simulink model "EGRVlv_VDSens"  (R2016b)
settings: configuration reference "CodeGenConfigSet" (kept outside this file)
values from neighbouring files (symbols this model uses):
  EGRVlv_facAdapClsStrt_C = Calibration.Parameter    [init_EGRVlv_VDSens.m]
  EGRVlv_facAdapPosCls_C = Calibration.Parameter    [init_EGRVlv_VDSens.m]
  EGRVlv_facPT1_C = Calibration.Parameter    [init_EGRVlv_VDSens.m]
  EGRVlv_facPT1ModVal_C = Calibration.Parameter    [init_EGRVlv_VDSens.m]
  EGRVlv_IKiOfsLrnUp_C = Calibration.Parameter    [init_EGRVlv_VDSens.m]
  EGRVlv_numAdapClsMax_C = Calibration.Parameter    [init_EGRVlv_VDSens.m]
  EGRVlv_numEngTempOfsLrnRls1_C = Calibration.Parameter    [init_EGRVlv_VDSens.m]
  EGRVlv_numEngTempOfsLrnRls2_C = Calibration.Parameter    [init_EGRVlv_VDSens.m]
  EGRVlv_numTempSel_C = Calibration.Parameter    [init_EGRVlv_VDSens.m]
  EGRVlv_rActMax_C = Calibration.Parameter    [init_EGRVlv_VDSens.m]
  EGRVlv_rActMin_C = Calibration.Parameter    [init_EGRVlv_VDSens.m]
  EGRVlv_rActOfs_C = Calibration.Parameter    [init_EGRVlv_VDSens.m]
  EGRVlv_rAdapAgOpnMax_C = Calibration.Parameter    [init_EGRVlv_VDSens.m]
  EGRVlv_rAdapAgOpnMin_C = Calibration.Parameter    [init_EGRVlv_VDSens.m]
  EGRVlv_rAdapDiffPlaus_C = Calibration.Parameter    [init_EGRVlv_VDSens.m]
  EGRVlv_rAdapDiffPlausLgT_C = Calibration.Parameter    [init_EGRVlv_VDSens.m]
  EGRVlv_rAdapDiffPlausShT_C = Calibration.Parameter    [init_EGRVlv_VDSens.m]
  EGRVlv_rAdapIniOpn0_C = Calibration.Parameter    [init_EGRVlv_VDSens.m]
  EGRVlv_rAdapIniOpn_C = Calibration.Parameter    [init_EGRVlv_VDSens.m]
  EGRVlv_rAdapOpnBnd_C = Calibration.Parameter    [init_EGRVlv_VDSens.m]
  EGRVlv_rCmpNewCtlUn_C = Calibration.Parameter    [init_EGRVlv_VDSens.m]
  EGRVlv_RmpSlpNeg_C = Calibration.Parameter    [init_EGRVlv_VDSens.m]
  EGRVlv_RmpSlpPos_C = Calibration.Parameter    [init_EGRVlv_VDSens.m]
  EGRVlv_rOfsLrnDwn_C = Calibration.Parameter    [init_EGRVlv_VDSens.m]
  EGRVlv_rOfsLrnRmpDwnCls_C = Calibration.Parameter    [init_EGRVlv_VDSens.m]
  EGRVlv_rOfsLrnRmpUpFst_C = Calibration.Parameter    [init_EGRVlv_VDSens.m]
  EGRVlv_rOfsLrnVlvMax_C = Calibration.Parameter    [init_EGRVlv_VDSens.m]
  EGRVlv_rOfsLrnVlvMin_C = Calibration.Parameter    [init_EGRVlv_VDSens.m]
  EGRVlv_rOfsMax_C = Calibration.Parameter    [init_EGRVlv_VDSens.m]
  EGRVlv_rOfsMin_C = Calibration.Parameter    [init_EGRVlv_VDSens.m]
  EGRVlv_rPullDwnThres_C = Calibration.Parameter    [init_EGRVlv_VDSens.m]
  EGRVlv_rRmpDwnCls_C = Calibration.Parameter    [init_EGRVlv_VDSens.m]
  EGRVlv_rRmpUpFst_C = Calibration.Parameter    [init_EGRVlv_VDSens.m]
  EGRVlv_rSensVlvThres_C = Calibration.Parameter    [init_EGRVlv_VDSens.m]
  EGRVlv_rTmpOfsLrnMax_C = Calibration.Parameter    [init_EGRVlv_VDSens.m]
  EGRVlv_rTmpOfsLrnMin_C = Calibration.Parameter    [init_EGRVlv_VDSens.m]
  EGRVlv_rTransStgDfl_C = Calibration.Parameter    [init_EGRVlv_VDSens.m]
  EGRVlv_stNewVlvTrg_C = Calibration.Parameter    [init_EGRVlv_VDSens.m]
  EGRVlv_stOfsEngCond_C = Calibration.Parameter    [init_EGRVlv_VDSens.m]
  EGRVlv_stOfsLrnEnb_C = Calibration.Parameter    [init_EGRVlv_VDSens.m]
  EGRVlv_stOfsLrnTrg_C = Calibration.Parameter    [init_EGRVlv_VDSens.m]
  EGRVlv_swtActOfs_C = Calibration.Parameter    [init_EGRVlv_VDSens.m]
  EGRVlv_swtOfsLrnActv_C = Calibration.Parameter    [init_EGRVlv_VDSens.m]
  EGRVlv_swtSensPrs_C = Calibration.Parameter    [init_EGRVlv_VDSens.m]
  EGRVlv_tEngFldThresOfsLrnRls1_C = Calibration.Parameter    [init_EGRVlv_VDSens.m]
  EGRVlv_tEngFldThresOfsLrnRls2_C = Calibration.Parameter    [init_EGRVlv_VDSens.m]
  EGRVlv_tEngMax_C = Calibration.Parameter    [init_EGRVlv_VDSens.m]
  EGRVlv_tEngMin_C = Calibration.Parameter    [init_EGRVlv_VDSens.m]
  EGRVlv_tiAdapJamVlv_C = Calibration.Parameter    [init_EGRVlv_VDSens.m]
  EGRVlv_tiAdapWaitSensAcq_C = Calibration.Parameter    [init_EGRVlv_VDSens.m]
  EGRVlv_tiClsJamVlv_C = Calibration.Parameter    [init_EGRVlv_VDSens.m]
  EGRVlv_tiStable_C = Calibration.Parameter    [init_EGRVlv_VDSens.m]
  EGRVlv_uBattMax_C = Calibration.Parameter    [init_EGRVlv_VDSens.m]
  EGRVlv_uBattMin_C = Calibration.Parameter    [init_EGRVlv_VDSens.m]
  PRC_ZERO = fi(0,Prc_100_rate)    [init_EGRVlv_VDSens.m]
  SigTst_rEGRVlv_C = Calibration.Parameter    [init_EGRVlv_VDSens.m]
  SigTst_swtEGRVlv_C = Calibration.Parameter    [init_EGRVlv_VDSens.m]
undefined symbols (not defined in the file or in its folder): CEngDst_switch_conv, EGRVlv_VDSens_DT, EngState_conv, SubSysExeState_conv, Switch_conv
libraries: simulink x22, CXLib x18
(part 1 of 2)
settings Model: Creator=lvzhanghui  LastModifiedBy=zhulinfeng
settings ConfigSetRef: SourceLocation=Base Workspace

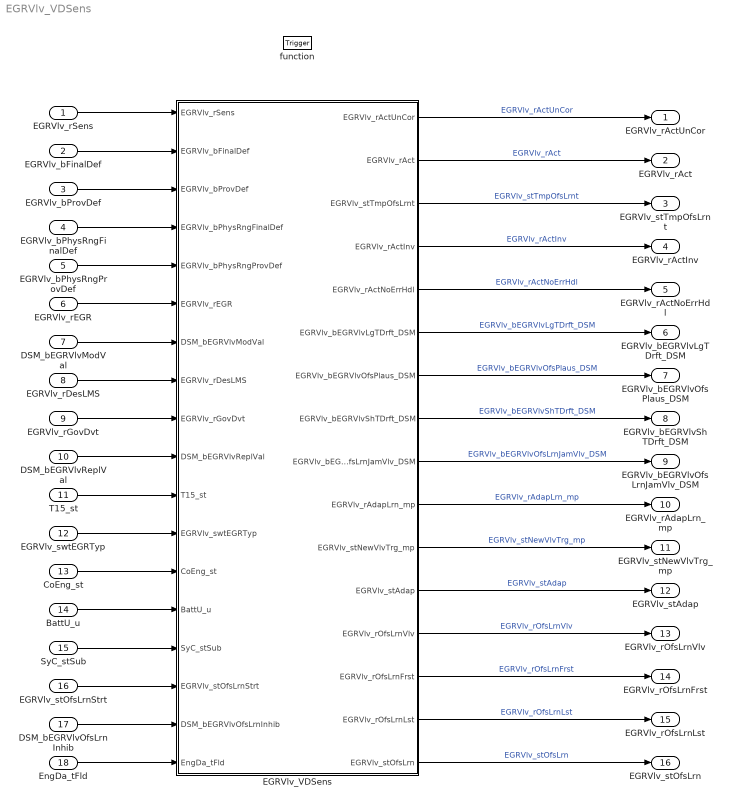
== system EGRVlv_VDSens ==
  EGRVlv_rSens : Inport  Tag=%  Description=Sensed value of actuator position without error handling  OutMin=-100  OutMax=100  OutDataTypeStr=Prc_100_rate
  EGRVlv_bFinalDef : Inport  Description=the final fault flag  Port=2  OutMin=0  OutMax=1  OutDataTypeStr=boolean
  EGRVlv_bProvDef : Inport  Description=the fault flag for the moment  Port=3  OutMin=0  OutMax=1  OutDataTypeStr=boolean
  EGRVlv_bPhysRngFinalDef : Inport  Description=Status Sensor of the EGR valve physical Signal range check finally defect  Port=4  OutMin=0  OutMax=1  OutDataTypeStr=boolean
  EGRVlv_bPhysRngProvDef : Inport  Description=Status Sensor of the EGR valve physical Signal range check temporary defect  Port=5  OutMin=0  OutMax=1  OutDataTypeStr=boolean
  EGRVlv_rEGR : Inport  Tag=%  Description=Control value for the EGR valve  Port=6  OutMin=-100  OutMax=100  OutDataTypeStr=Prc_100_rate
  DSM_bEGRVlvModVal : Inport  Description=Status of FId_EGRVlvModVal  Port=7  OutMin=0  OutMax=1  OutDataTypeStr=boolean
  EGRVlv_rDesLMS : Inport  Tag=%  Description=Desired value from LMS control  Port=8  OutMin=-100  OutMax=100  OutDataTypeStr=Prc_100_rate
  EGRVlv_rGovDvt : Inport  Tag=%  Description=Control deviation  Port=9  OutMin=-100  OutMax=100  OutDataTypeStr=Prc_100_rate
  DSM_bEGRVlvReplVal : Inport  Description=Status of FId_EGRVlvReplVal  Port=10  OutMin=0  OutMax=1  OutDataTypeStr=boolean
  T15_st : Inport  Description=Terminal 15 status after denouncing  Port=11  OutDataTypeStr=Enum: Switch_conv
  EGRVlv_swtEGRTyp : Inport  Description=Type of EGR actuator used  Port=12  OutMin=0  OutMax=255  OutDataTypeStr=State_uint8
  CoEng_st : Inport  Description=Engine coordinator state  Port=13  OutDataTypeStr=Enum: EngState_conv
  BattU_u : Inport  Tag=mv  Description=Battery voltage  Port=14  OutMin=0  OutMax=50000  OutDataTypeStr=Battery_mv
  SyC_stSub : Inport  Description=Current system/ECU sub-state  Port=15  OutDataTypeStr=Enum: SubSysExeState_conv
  EGRVlv_stOfsLrnStrt : Inport  Description=Diagnosis tester value to start offset learning  Port=16  OutMin=0  OutMax=1  OutDataTypeStr=boolean
  DSM_bEGRVlvOfsLrnInhib : Inport  Description=FId inhibited in case of system fault  Port=17  OutMin=0  OutMax=1  OutDataTypeStr=boolean
  EngDa_tFld : Inport  Tag=deg  Description=Engine temperature field  Port=18  OutMin=-3000  OutMax=3000  OutDataTypeStr=Temp_deg  PortDimensions=3
  function : TriggerPort  TriggerType=function-call  VariantControl=Variant
  EGRVlv_VDSens : Subsystem
  EGRVlv_rActUnCor : Outport  Tag=%  Description=Uncorrected position of the valve  OutMin=-100  OutMax=100  OutDataTypeStr=Prc_100_rate
  EGRVlv_rAct : Outport  Tag=%  Description=Actuatorposition  Port=2  OutMin=-100  OutMax=100  OutDataTypeStr=Prc_100_rate
  EGRVlv_stTmpOfsLrnt : Outport  Description=Temporary offset of the EGR valve is already learnt in the current driving cycle  Port=3  OutMin=0  OutMax=1  OutDataTypeStr=boolean
  EGRVlv_rActInv : Outport  Tag=%  Description=Actuatorposition (100% - rAct)  Port=4  OutMin=-100  OutMax=100  OutDataTypeStr=Prc_100_rate
  EGRVlv_rActNoErrHdl : Outport  Tag=%  Description=Valve position (offset corrected without error handling)  Port=5  OutMin=-100  OutMax=100  OutDataTypeStr=Prc_100_rate
  EGRVlv_bEGRVlvLgTDrft_DSM : Outport  Description=Fault path for long time valve drift  Port=6  OutMin=0  OutMax=1  OutDataTypeStr=boolean
  EGRVlv_bEGRVlvOfsPlaus_DSM : Outport  Description=Fault path for plausibility error  Port=7  OutMin=0  OutMax=1  OutDataTypeStr=boolean
  EGRVlv_bEGRVlvShTDrft_DSM : Outport  Description=Fault path for short time valve drift  Port=8  OutMin=0  OutMax=1  OutDataTypeStr=boolean
  EGRVlv_bEGRVlvOfsLrnJamVlv_DSM : Outport  Description=Fault path for jammed valve error during offset learning  Port=9  OutMin=0  OutMax=1  OutDataTypeStr=boolean
  EGRVlv_rAdapLrn_mp : Outport  Tag=%  Description=Offset learnt value in the present driving cycle  Port=10  OutMin=-100  OutMax=100  OutDataTypeStr=Prc_100_rate
  EGRVlv_stNewVlvTrg_mp : Outport  Description=New valve trigger status  Port=11  OutMin=0  OutMax=1  OutDataTypeStr=boolean
  EGRVlv_stAdap : Outport  Description=Status of offset learning  Port=12  OutMin=0  OutMax=65535  OutDataTypeStr=State_uint16
  EGRVlv_rOfsLrnVlv : Outport  Tag=%  Description=Control value for offset learning  Port=13  OutMin=-100  OutMax=100  OutDataTypeStr=Prc_100_rate
  EGRVlv_rOfsLrnFrst : Outport  Tag=%  Description=First learnt offset value stored in EEPROM  Port=14  OutMin=-100  OutMax=100  OutDataTypeStr=Prc_100_rate
  EGRVlv_rOfsLrnLst : Outport  Tag=%  Description=Last learnt offset value stored in EEPROM  Port=15  OutMin=-100  OutMax=100  OutDataTypeStr=Prc_100_rate
  EGRVlv_stOfsLrn : Outport  Description=Offset learning for Throttle valve complete  Port=16  OutMin=0  OutMax=255  OutDataTypeStr=State_uint8
  wires:
  EGRVlv_rSens/1 -> EGRVlv_VDSens/1(EGRVlv_rSens)
  EGRVlv_bFinalDef/1 -> EGRVlv_VDSens/2(EGRVlv_bFinalDef)
  EGRVlv_bProvDef/1 -> EGRVlv_VDSens/3(EGRVlv_bProvDef)
  EGRVlv_bPhysRngFinalDef/1 -> EGRVlv_VDSens/4(EGRVlv_bPhysRngFinalDef)
  EGRVlv_bPhysRngProvDef/1 -> EGRVlv_VDSens/5(EGRVlv_bPhysRngProvDef)
  EGRVlv_rEGR/1 -> EGRVlv_VDSens/6(EGRVlv_rEGR)
  DSM_bEGRVlvModVal/1 -> EGRVlv_VDSens/7(DSM_bEGRVlvModVal)
  EGRVlv_rDesLMS/1 -> EGRVlv_VDSens/8(EGRVlv_rDesLMS)
  EGRVlv_rGovDvt/1 -> EGRVlv_VDSens/9(EGRVlv_rGovDvt)
  DSM_bEGRVlvReplVal/1 -> EGRVlv_VDSens/10(DSM_bEGRVlvReplVal)
  T15_st/1 -> EGRVlv_VDSens/11(T15_st)
  EGRVlv_swtEGRTyp/1 -> EGRVlv_VDSens/12(EGRVlv_swtEGRTyp)
  CoEng_st/1 -> EGRVlv_VDSens/13(CoEng_st)
  BattU_u/1 -> EGRVlv_VDSens/14(BattU_u)
  SyC_stSub/1 -> EGRVlv_VDSens/15(SyC_stSub)
  EGRVlv_stOfsLrnStrt/1 -> EGRVlv_VDSens/16(EGRVlv_stOfsLrnStrt)
  DSM_bEGRVlvOfsLrnInhib/1 -> EGRVlv_VDSens/17(DSM_bEGRVlvOfsLrnInhib)
  EngDa_tFld/1 -> EGRVlv_VDSens/18(EngDa_tFld)
  EGRVlv_VDSens/1(EGRVlv_rActUnCor) -> EGRVlv_rActUnCor/1  "EGRVlv_rActUnCor"
  EGRVlv_VDSens/2(EGRVlv_rAct) -> EGRVlv_rAct/1  "EGRVlv_rAct"
  EGRVlv_VDSens/3(EGRVlv_stTmpOfsLrnt) -> EGRVlv_stTmpOfsLrnt/1  "EGRVlv_stTmpOfsLrnt"
  EGRVlv_VDSens/4(EGRVlv_rActInv) -> EGRVlv_rActInv/1  "EGRVlv_rActInv"
  EGRVlv_VDSens/5(EGRVlv_rActNoErrHdl) -> EGRVlv_rActNoErrHdl/1  "EGRVlv_rActNoErrHdl"
  EGRVlv_VDSens/6(EGRVlv_bEGRVlvLgTDrft_DSM) -> EGRVlv_bEGRVlvLgTDrft_DSM/1  "EGRVlv_bEGRVlvLgTDrft_DSM"
  EGRVlv_VDSens/7(EGRVlv_bEGRVlvOfsPlaus_DSM) -> EGRVlv_bEGRVlvOfsPlaus_DSM/1  "EGRVlv_bEGRVlvOfsPlaus_DSM"
  EGRVlv_VDSens/8(EGRVlv_bEGRVlvShTDrft_DSM) -> EGRVlv_bEGRVlvShTDrft_DSM/1  "EGRVlv_bEGRVlvShTDrft_DSM"
  EGRVlv_VDSens/9(EGRVlv_bEGRVlvOfsLrnJamVlv_DSM) -> EGRVlv_bEGRVlvOfsLrnJamVlv_DSM/1  "EGRVlv_bEGRVlvOfsLrnJamVlv_DSM"
  EGRVlv_VDSens/10(EGRVlv_rAdapLrn_mp) -> EGRVlv_rAdapLrn_mp/1  "EGRVlv_rAdapLrn_mp"
  EGRVlv_VDSens/11(EGRVlv_stNewVlvTrg_mp) -> EGRVlv_stNewVlvTrg_mp/1  "EGRVlv_stNewVlvTrg_mp"
  EGRVlv_VDSens/12(EGRVlv_stAdap) -> EGRVlv_stAdap/1  "EGRVlv_stAdap"
  EGRVlv_VDSens/13(EGRVlv_rOfsLrnVlv) -> EGRVlv_rOfsLrnVlv/1  "EGRVlv_rOfsLrnVlv"
  EGRVlv_VDSens/16(EGRVlv_stOfsLrn) -> EGRVlv_stOfsLrn/1  "EGRVlv_stOfsLrn"
  EGRVlv_VDSens/14(EGRVlv_rOfsLrnFrst) -> EGRVlv_rOfsLrnFrst/1  "EGRVlv_rOfsLrnFrst"
  EGRVlv_VDSens/15(EGRVlv_rOfsLrnLst) -> EGRVlv_rOfsLrnLst/1  "EGRVlv_rOfsLrnLst"

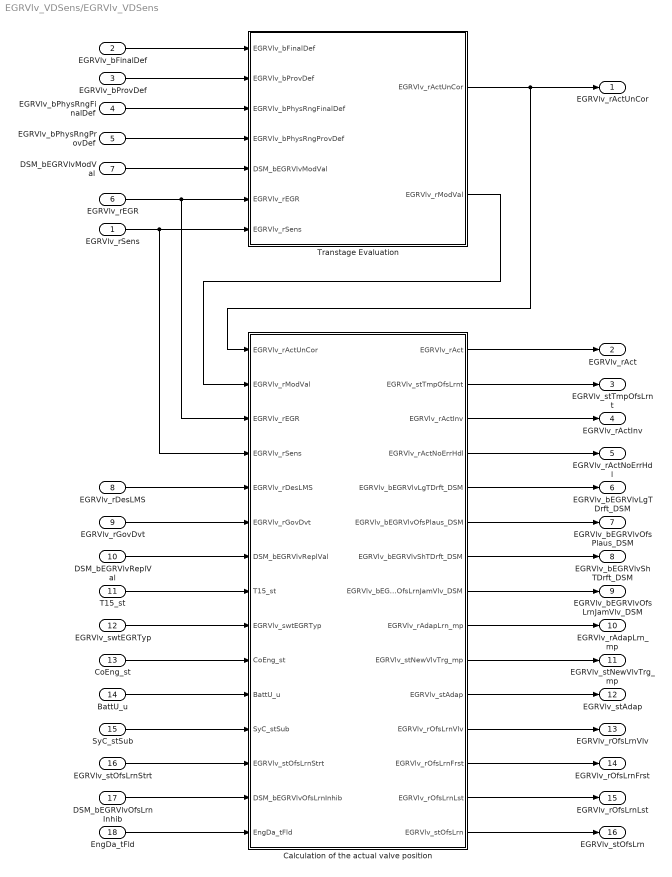
== system EGRVlv_VDSens/EGRVlv_VDSens ==
  EGRVlv_rSens : Inport  Tag=%
  EGRVlv_bFinalDef : Inport  Port=2
  EGRVlv_bProvDef : Inport  Port=3
  EGRVlv_bPhysRngFinalDef : Inport  Port=4
  EGRVlv_bPhysRngProvDef : Inport  Port=5
  EGRVlv_rEGR : Inport  Tag=%  Port=6
  DSM_bEGRVlvModVal : Inport  Tag=%  Port=7
  EGRVlv_rDesLMS : Inport  Port=8
  EGRVlv_rGovDvt : Inport  Port=9
  DSM_bEGRVlvReplVal : Inport  Tag=%  Port=10
  T15_st : Inport  Tag=%  Port=11
  EGRVlv_swtEGRTyp : Inport  Tag=%  Port=12
  CoEng_st : Inport  Port=13
  BattU_u : Inport  Tag=%  Port=14
  SyC_stSub : Inport  Tag=%  Port=15
  EGRVlv_stOfsLrnStrt : Inport  Tag=%  Port=16
  DSM_bEGRVlvOfsLrnInhib : Inport  Port=17
  EngDa_tFld : Inport  Tag=%  Port=18
  Calculation of the actual valve position : Subsystem
  Transtage Evaluation : Subsystem
  EGRVlv_rActUnCor : Outport  Tag=%
  EGRVlv_rAct : Outport  Tag=%  Port=2
  EGRVlv_stTmpOfsLrnt : Outport  Port=3
  EGRVlv_rActInv : Outport  Tag=%  Port=4
  EGRVlv_rActNoErrHdl : Outport  Port=5
  EGRVlv_bEGRVlvLgTDrft_DSM : Outport  Port=6
  EGRVlv_bEGRVlvOfsPlaus_DSM : Outport  Port=7
  EGRVlv_bEGRVlvShTDrft_DSM : Outport  Port=8
  EGRVlv_bEGRVlvOfsLrnJamVlv_DSM : Outport  Tag=%  Port=9
  EGRVlv_rAdapLrn_mp : Outport  Tag=%  Port=10
  EGRVlv_stNewVlvTrg_mp : Outport  Port=11
  EGRVlv_stAdap : Outport  Port=12
  EGRVlv_rOfsLrnVlv : Outport  Port=13
  EGRVlv_rOfsLrnFrst : Outport  Port=14
  EGRVlv_rOfsLrnLst : Outport  Port=15
  EGRVlv_stOfsLrn : Outport  Tag=%  Port=16
  wires:
  Transtage Evaluation/1(EGRVlv_rActUnCor) -> EGRVlv_rActUnCor/1, Calculation of the actual valve position/1(EGRVlv_rActUnCor)
  EGRVlv_rSens/1 -> Calculation of the actual valve position/4(EGRVlv_rSens), Transtage Evaluation/7(EGRVlv_rSens)
  EGRVlv_rEGR/1 -> Calculation of the actual valve position/3(EGRVlv_rEGR), Transtage Evaluation/6(EGRVlv_rEGR)
  Transtage Evaluation/2(EGRVlv_rModVal) -> Calculation of the actual valve position/2(EGRVlv_rModVal)
  EGRVlv_rDesLMS/1 -> Calculation of the actual valve position/5(EGRVlv_rDesLMS)
  EGRVlv_rGovDvt/1 -> Calculation of the actual valve position/6(EGRVlv_rGovDvt)
  DSM_bEGRVlvReplVal/1 -> Calculation of the actual valve position/7(DSM_bEGRVlvReplVal)
  T15_st/1 -> Calculation of the actual valve position/8(T15_st)
  EGRVlv_swtEGRTyp/1 -> Calculation of the actual valve position/9(EGRVlv_swtEGRTyp)
  CoEng_st/1 -> Calculation of the actual valve position/10(CoEng_st)
  BattU_u/1 -> Calculation of the actual valve position/11(BattU_u)
  SyC_stSub/1 -> Calculation of the actual valve position/12(SyC_stSub)
  EGRVlv_stOfsLrnStrt/1 -> Calculation of the actual valve position/13(EGRVlv_stOfsLrnStrt)
  DSM_bEGRVlvOfsLrnInhib/1 -> Calculation of the actual valve position/14(DSM_bEGRVlvOfsLrnInhib)
  EngDa_tFld/1 -> Calculation of the actual valve position/15(EngDa_tFld)
  EGRVlv_bFinalDef/1 -> Transtage Evaluation/1(EGRVlv_bFinalDef)
  EGRVlv_bProvDef/1 -> Transtage Evaluation/2(EGRVlv_bProvDef)
  EGRVlv_bPhysRngFinalDef/1 -> Transtage Evaluation/3(EGRVlv_bPhysRngFinalDef)
  EGRVlv_bPhysRngProvDef/1 -> Transtage Evaluation/4(EGRVlv_bPhysRngProvDef)
  DSM_bEGRVlvModVal/1 -> Transtage Evaluation/5(DSM_bEGRVlvModVal)
  Calculation of the actual valve position/1(EGRVlv_rAct) -> EGRVlv_rAct/1
  Calculation of the actual valve position/2(EGRVlv_stTmpOfsLrnt) -> EGRVlv_stTmpOfsLrnt/1
  Calculation of the actual valve position/3(EGRVlv_rActInv) -> EGRVlv_rActInv/1
  Calculation of the actual valve position/4(EGRVlv_rActNoErrHdl) -> EGRVlv_rActNoErrHdl/1
  Calculation of the actual valve position/5(EGRVlv_bEGRVlvLgTDrft_DSM) -> EGRVlv_bEGRVlvLgTDrft_DSM/1
  Calculation of the actual valve position/6(EGRVlv_bEGRVlvOfsPlaus_DSM) -> EGRVlv_bEGRVlvOfsPlaus_DSM/1
  Calculation of the actual valve position/7(EGRVlv_bEGRVlvShTDrft_DSM) -> EGRVlv_bEGRVlvShTDrft_DSM/1
  Calculation of the actual valve position/8(EGRVlv_bEGRVlvOfsLrnJamVlv_DSM) -> EGRVlv_bEGRVlvOfsLrnJamVlv_DSM/1
  Calculation of the actual valve position/9(EGRVlv_rAdapLrn_mp) -> EGRVlv_rAdapLrn_mp/1
  Calculation of the actual valve position/10(EGRVlv_stNewVlvTrg_mp) -> EGRVlv_stNewVlvTrg_mp/1
  Calculation of the actual valve position/11(EGRVlv_stAdap) -> EGRVlv_stAdap/1
  Calculation of the actual valve position/12(EGRVlv_rOfsLrnVlv) -> EGRVlv_rOfsLrnVlv/1
  Calculation of the actual valve position/13(EGRVlv_rOfsLrnFrst) -> EGRVlv_rOfsLrnFrst/1
  Calculation of the actual valve position/14(EGRVlv_rOfsLrnLst) -> EGRVlv_rOfsLrnLst/1
  Calculation of the actual valve position/15(EGRVlv_stOfsLrn) -> EGRVlv_stOfsLrn/1

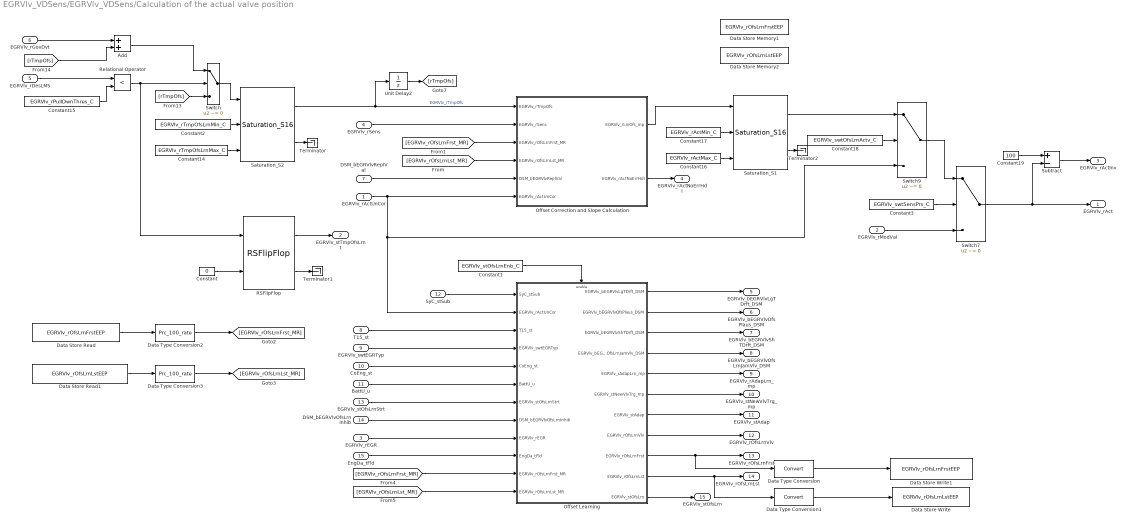
== system EGRVlv_VDSens/EGRVlv_VDSens/Calculation of the actual valve position ==
  EGRVlv_rActUnCor : Inport  Tag=%
  EGRVlv_rModVal : Inport  Tag=%  Port=2
  EGRVlv_rEGR : Inport  Tag=%  Port=3
  EGRVlv_rSens : Inport  Tag=%  Port=4
  EGRVlv_rDesLMS : Inport  Port=5
  EGRVlv_rGovDvt : Inport  Port=6
  DSM_bEGRVlvReplVal : Inport  Tag=%  Port=7
  T15_st : Inport  Tag=%  Port=8
  EGRVlv_swtEGRTyp : Inport  Tag=%  Port=9
  CoEng_st : Inport  Port=10
  BattU_u : Inport  Tag=%  Port=11
  SyC_stSub : Inport  Tag=%  Port=12
  EGRVlv_stOfsLrnStrt : Inport  Tag=%  Port=13
  DSM_bEGRVlvOfsLrnInhib : Inport  Port=14
  EngDa_tFld : Inport  Tag=%  Port=15
  Add : Sum  SaturateOnIntegerOverflow=on
  Constant : Constant  Value=0  OutDataTypeStr=boolean
  Constant1 : Constant  Value=EGRVlv_stOfsLrnEnb_C
  Constant14 : Constant  Value=EGRVlv_rTmpOfsLrnMax_C  SampleTime=-1
  Constant15 : Constant  Value=EGRVlv_rPullDwnThres_C  SampleTime=-1
  Constant16 : Constant  Value=EGRVlv_rActMax_C  SampleTime=-1
  Constant17 : Constant  Value=EGRVlv_rActMin_C  SampleTime=-1
  Constant18 : Constant  Value=EGRVlv_swtOfsLrnActv_C  SampleTime=-1
  Constant19 : Constant  Value=100  OutDataTypeStr=Prc_100_rate
  Constant2 : Constant  Value=EGRVlv_rTmpOfsLrnMin_C  SampleTime=-1
  Constant3 : Constant  Value=EGRVlv_swtSensPrs_C
  Data Store Memory1 : DataStoreMemory  DataStoreName=EGRVlv_rOfsLrnFrstEEP  ReadBeforeWriteMsg=warning  WriteAfterWriteMsg=warning  WriteAfterReadMsg=warning  ShowAdditionalParam=off  OutDataTypeStr=fixdt(1,16,100/8192,0)
  Data Store Memory2 : DataStoreMemory  DataStoreName=EGRVlv_rOfsLrnLstEEP  ReadBeforeWriteMsg=warning  WriteAfterWriteMsg=warning  WriteAfterReadMsg=warning  ShowAdditionalParam=off  OutDataTypeStr=fixdt(1,16,100/8192,0)
  Data Store Read : DataStoreRead  DataStoreName=EGRVlv_rOfsLrnFrstEEP
  Data Store Read1 : DataStoreRead  DataStoreName=EGRVlv_rOfsLrnLstEEP
  Data Store Write : DataStoreWrite  DataStoreName=EGRVlv_rOfsLrnLstEEP
  Data Store Write1 : DataStoreWrite  DataStoreName=EGRVlv_rOfsLrnFrstEEP
  Data Type Conversion : DataTypeConversion
  Data Type Conversion1 : DataTypeConversion
  Data Type Conversion2 : DataTypeConversion  OutDataTypeStr=Prc_100_rate
  Data Type Conversion3 : DataTypeConversion  OutDataTypeStr=Prc_100_rate
  Offset Correction and Slope Calculation : Subsystem
  Offset Learning : Subsystem
  RSFlipFlop : CXLib/RSFlipFlop
  Relational Operator : RelationalOperator  Operator=<  OutDataTypeStr=boolean  RndMeth=Simplest
  Saturation_S1 : CXLib/Saturation_S16
  Saturation_S2 : CXLib/Saturation_S16
  Subtract : Sum  Inputs=+-  SaturateOnIntegerOverflow=on
  Switch : Switch  Criteria=u2 ~= 0
  Switch7 : Switch  Criteria=u2 ~= 0  Threshold=CEngDst_switch_conv.OFF  InputSameDT=on
  Switch9 : Switch  Criteria=u2 ~= 0  Threshold=CEngDst_switch_conv.OFF  InputSameDT=on
  Terminator : Terminator
  Terminator1 : Terminator
  Terminator2 : Terminator
  Unit Delay2 : UnitDelay  SampleTime=-1
      settings: AttributesFormatString=InitialValue=%<InitialCondition>
  EGRVlv_rAct : Outport  Tag=%
  EGRVlv_stTmpOfsLrnt : Outport  Port=2
  EGRVlv_rActInv : Outport  Tag=%  Port=3
  EGRVlv_rActNoErrHdl : Outport  Port=4
  EGRVlv_bEGRVlvLgTDrft_DSM : Outport  Port=5
  EGRVlv_bEGRVlvOfsPlaus_DSM : Outport  Port=6
  EGRVlv_bEGRVlvShTDrft_DSM : Outport  Port=7
  EGRVlv_bEGRVlvOfsLrnJamVlv_DSM : Outport  Tag=%  Port=8
  EGRVlv_rAdapLrn_mp : Outport  Tag=%  Port=9
  EGRVlv_stNewVlvTrg_mp : Outport  Port=10
  EGRVlv_stAdap : Outport  Port=11
  EGRVlv_rOfsLrnVlv : Outport  Port=12
  EGRVlv_rOfsLrnFrst : Outport  Port=13
  EGRVlv_rOfsLrnLst : Outport  Port=14
  EGRVlv_stOfsLrn : Outport  Tag=%  Port=15
  wires:
  Constant3/1 -> Switch7/2
  Switch7/1 -> EGRVlv_rAct/1, Subtract/2
  Constant14/1 -> Saturation_S2/3
  Constant2/1 -> Saturation_S2/2
  Constant15/1 -> Relational Operator/2
  EGRVlv_rDesLMS/1 -> Relational Operator/1
  Relational Operator/1 -> RSFlipFlop/1, Switch/2
  EGRVlv_rGovDvt/1 -> Add/1
  Add/1 -> Switch/1
  [rTmpOfs] -> Switch/3
  Switch/1 -> Saturation_S2/1
  Saturation_S2/1 -> Offset Correction and Slope Calculation/1(EGRVlv_rTmpOfs), Unit Delay2/1  "EGRVlv_rTmpOfs"
  [rTmpOfs] -> Add/2
  Constant/1 -> RSFlipFlop/2
  Constant16/1 -> Saturation_S1/3
  Saturation_S1/1 -> Switch9/1
  Constant18/1 -> Switch9/2
  Constant17/1 -> Saturation_S1/2
  Switch9/1 -> Switch7/1
  Offset Correction and Slope Calculation/1(EGRVlv_rLinOfs_mp) -> Saturation_S1/1
  Constant19/1 -> Subtract/1
  Subtract/1 -> EGRVlv_rActInv/1
  Unit Delay2/1 -> [rTmpOfs]
  EGRVlv_rModVal/1 -> Switch7/3
  EGRVlv_rActUnCor/1 -> Offset Correction and Slope Calculation/6(EGRVlv_rActUnCor), Offset Learning/2(EGRVlv_rActUnCor), Switch9/3
  SyC_stSub/1 -> Offset Learning/1(SyC_stSub)
  EGRVlv_rSens/1 -> Offset Correction and Slope Calculation/2(EGRVlv_rSens)
  DSM_bEGRVlvReplVal/1 -> Offset Correction and Slope Calculation/5(DSM_bEGRVlvReplVal)
  T15_st/1 -> Offset Learning/3(T15_st)
  EGRVlv_swtEGRTyp/1 -> Offset Learning/4(EGRVlv_swtEGRTyp)
  CoEng_st/1 -> Offset Learning/5(CoEng_st)
  BattU_u/1 -> Offset Learning/6(BattU_u)
  EGRVlv_stOfsLrnStrt/1 -> Offset Learning/7(EGRVlv_stOfsLrnStrt)
  DSM_bEGRVlvOfsLrnInhib/1 -> Offset Learning/8(DSM_bEGRVlvOfsLrnInhib)
  EGRVlv_rEGR/1 -> Offset Learning/9(EGRVlv_rEGR)
  EngDa_tFld/1 -> Offset Learning/10(EngDa_tFld)
  [EGRVlv_rOfsLrnFrst_MR] -> Offset Learning/11(EGRVlv_rOfsLrnFrst_MR)
  [EGRVlv_rOfsLrnLst_MR] -> Offset Learning/12(EGRVlv_rOfsLrnLst_MR)
  Offset Correction and Slope Calculation/2(EGRVlv_rActNoErrHdl) -> EGRVlv_rActNoErrHdl/1
  Offset Learning/1(EGRVlv_bEGRVlvLgTDrft_DSM) -> EGRVlv_bEGRVlvLgTDrft_DSM/1
  Offset Learning/2(EGRVlv_bEGRVlvOfsPlaus_DSM) -> EGRVlv_bEGRVlvOfsPlaus_DSM/1
  Offset Learning/3(EGRVlv_bEGRVlvShTDrft_DSM) -> EGRVlv_bEGRVlvShTDrft_DSM/1
  Offset Learning/4(EGRVlv_bEGRVlvOfsLrnJamVlv_DSM) -> EGRVlv_bEGRVlvOfsLrnJamVlv_DSM/1
  Offset Learning/5(EGRVlv_rAdapLrn_mp) -> EGRVlv_rAdapLrn_mp/1
  Offset Learning/6(EGRVlv_stNewVlvTrg_mp) -> EGRVlv_stNewVlvTrg_mp/1
  Offset Learning/7(EGRVlv_stAdap) -> EGRVlv_stAdap/1
  Offset Learning/8(EGRVlv_rOfsLrnVlv) -> EGRVlv_rOfsLrnVlv/1
  RSFlipFlop/1 -> EGRVlv_stTmpOfsLrnt/1
  RSFlipFlop/2 -> Terminator1/1
  Saturation_S1/2 -> Terminator2/1
  Saturation_S2/2 -> Terminator/1
  Offset Learning/11(EGRVlv_stOfsLrn) -> EGRVlv_stOfsLrn/1
  Constant1/1 -> Offset Learning/Enable
  [EGRVlv_rOfsLrnLst_MR] -> Offset Correction and Slope Calculation/4(EGRVlv_rOfsLrnLst_MR)
  [EGRVlv_rOfsLrnFrst_MR] -> Offset Correction and Slope Calculation/3(EGRVlv_rOfsLrnFrst_MR)
  Data Store Read/1 -> Data Type Conversion2/1
  Data Store Read1/1 -> Data Type Conversion3/1
  Offset Learning/10(EGRVlv_rOfsLrnLst) -> Data Type Conversion1/1, EGRVlv_rOfsLrnLst/1
  Offset Learning/9(EGRVlv_rOfsLrnFrst) -> Data Type Conversion/1, EGRVlv_rOfsLrnFrst/1
  Data Type Conversion/1 -> Data Store Write1/1
  Data Type Conversion1/1 -> Data Store Write/1
  Data Type Conversion2/1 -> [EGRVlv_rOfsLrnFrst_MR]
  Data Type Conversion3/1 -> [EGRVlv_rOfsLrnLst_MR]

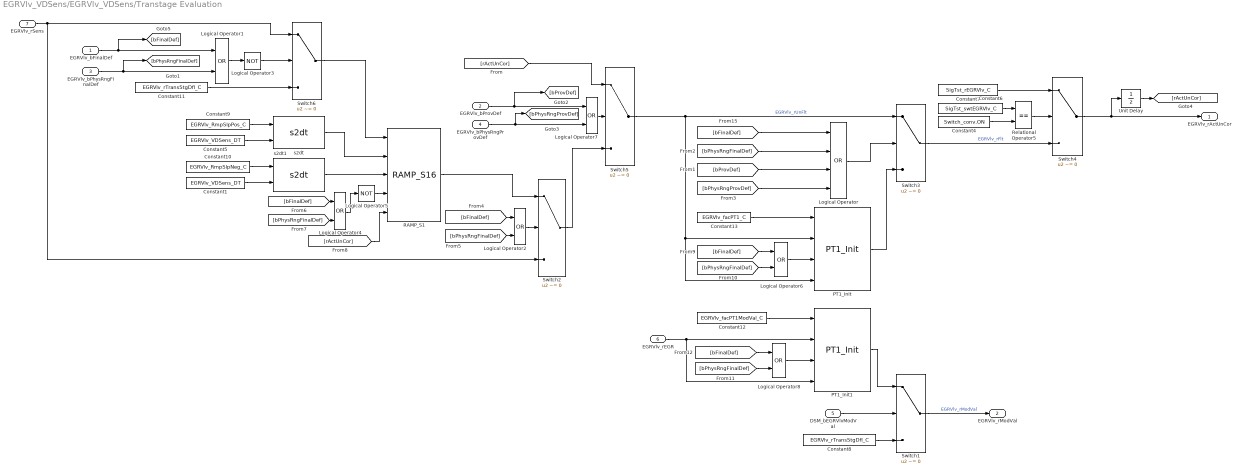
== system EGRVlv_VDSens/EGRVlv_VDSens/Transtage Evaluation ==
  EGRVlv_bFinalDef : Inport
  EGRVlv_bProvDef : Inport  Port=2
  EGRVlv_bPhysRngFinalDef : Inport  Port=3
  EGRVlv_bPhysRngProvDef : Inport  Port=4
  DSM_bEGRVlvModVal : Inport  Tag=%  Port=5
  EGRVlv_rEGR : Inport  Tag=%  Port=6
  EGRVlv_rSens : Inport  Tag=%  Port=7
  Constant1 : Constant  Value=EGRVlv_VDSens_DT
  Constant10 : Constant  Value=EGRVlv_RmpSlpNeg_C  SampleTime=-1
  Constant11 : Constant  Value=EGRVlv_rTransStgDfl_C  SampleTime=-1
  Constant12 : Constant  Value=EGRVlv_facPT1ModVal_C
  Constant13 : Constant  Value=EGRVlv_facPT1_C  SampleTime=-1
  Constant4 : Constant  Value=Switch_conv.ON
  Constant5 : Constant  Value=EGRVlv_VDSens_DT
  Constant6 : Constant  Value=SigTst_swtEGRVlv_C  SampleTime=-1
  Constant7 : Constant  Value=SigTst_rEGRVlv_C  SampleTime=-1
  Constant8 : Constant  Value=EGRVlv_rTransStgDfl_C
  Constant9 : Constant  Value=EGRVlv_RmpSlpPos_C  SampleTime=-1
  Logical Operator : Logic  Operator=OR  Inputs=4  OutDataTypeStr=boolean
  Logical Operator{1..2,4,6..8} (6 alike) : Logic  Operator=OR  OutDataTypeStr=boolean
  Logical Operator3 : Logic  Operator=NOT  AllPortsSameDT=off  OutDataTypeStr=boolean
  Logical Operator5 : Logic  Operator=NOT  AllPortsSameDT=off  OutDataTypeStr=boolean
  PT1_Init : CXLib/PT1_Init
  PT1_Init1 : CXLib/PT1_Init
  RAMP_S1 : CXLib/RAMP_S16
  Relational Operator5 : RelationalOperator  Operator===  OutDataTypeStr=boolean  RndMeth=Simplest  InputSameDT=on
  Switch1 : Switch  Criteria=u2 ~= 0  Threshold=CEngDst_switch_conv.OFF  InputSameDT=on
  Switch{2..3,5..6} (4 alike) : Switch  Criteria=u2 ~= 0  InputSameDT=on
  Switch4 : Switch  Criteria=u2 ~= 0  Threshold=CEngDst_switch_conv.OFF  InputSameDT=on
  Unit Delay : UnitDelay  SampleTime=-1
      settings: AttributesFormatString=InitialValue=%<InitialCondition>
  s2dt : CXLib/s2dt
  s2dt1 : CXLib/s2dt
  EGRVlv_rActUnCor : Outport  Tag=%
  EGRVlv_rModVal : Outport  Tag=%  Port=2
  wires:
  Constant6/1 -> Relational Operator5/1
  Logical Operator1/1 -> Logical Operator3/1
  Logical Operator3/1 -> Switch6/2
  Relational Operator5/1 -> Switch4/2
  [bPhysRngProvDef] -> Logical Operator/4
  [bPhysRngFinalDef] -> Logical Operator4/2
  Logical Operator5/1 -> RAMP_S1/4
  [rActUnCor] -> Switch5/1
  [bPhysRngFinalDef] -> Logical Operator6/2
  Constant5/1 -> s2dt/2
  [bFinalDef] -> Logical Operator2/1
  [bFinalDef] -> Logical Operator6/1
  Constant4/1 -> Relational Operator5/2
  s2dt1/1 -> RAMP_S1/3
  [bPhysRngFinalDef] -> Logical Operator2/2
  [bProvDef] -> Logical Operator/3
  s2dt/1 -> RAMP_S1/2
  [bPhysRngFinalDef] -> Logical Operator/2
  Logical Operator6/1 -> PT1_Init/3
  Constant1/1 -> s2dt1/2
  RAMP_S1/1 -> Switch2/1
  PT1_Init/1 -> Switch3/3
  Constant9/1 -> s2dt/1
  EGRVlv_bPhysRngProvDef/1 -> Logical Operator7/2, [bPhysRngProvDef]
  Logical Operator7/1 -> Switch5/2
  Logical Operator2/1 -> Switch2/2
  Logical Operator4/1 -> Logical Operator5/1
  Constant7/1 -> Switch4/1
  Switch6/1 -> RAMP_S1/1
  [bFinalDef] -> Logical Operator/1
  Unit Delay/1 -> [rActUnCor]
  EGRVlv_bFinalDef/1 -> Logical Operator1/1, [bFinalDef]
  Constant10/1 -> s2dt1/1
  EGRVlv_bPhysRngFinalDef/1 -> Logical Operator1/2, [bPhysRngFinalDef]
  Constant13/1 -> PT1_Init/1
  [bFinalDef] -> Logical Operator4/1
  EGRVlv_bProvDef/1 -> Logical Operator7/1, [bProvDef]
  Logical Operator/1 -> Switch3/2
  Constant11/1 -> Switch6/3
  EGRVlv_rSens/1 -> Switch6/1, Switch2/3
  Switch5/1 -> Switch3/1, PT1_Init/2, PT1_Init/4  "EGRVlv_rUnFlt"
  Switch3/1 -> Switch4/3  "EGRVlv_rFlt"
  Switch4/1 -> Unit Delay/1, EGRVlv_rActUnCor/1
  Switch2/1 -> Switch5/3
  DSM_bEGRVlvModVal/1 -> Switch1/2
  Switch1/1 -> EGRVlv_rModVal/1  "EGRVlv_rModVal"
  Constant8/1 -> Switch1/3
  PT1_Init1/1 -> Switch1/1
  EGRVlv_rEGR/1 -> PT1_Init1/2, PT1_Init1/4
  Constant12/1 -> PT1_Init1/1
  [bPhysRngFinalDef] -> Logical Operator8/2
  [bFinalDef] -> Logical Operator8/1
  Logical Operator8/1 -> PT1_Init1/3
  [rActUnCor] -> RAMP_S1/5

== system EGRVlv_VDSens/EGRVlv_VDSens/Calculation of the actual valve position/Offset Correction and Slope Calculation ==
  EGRVlv_rTmpOfs : Inport  Tag=%
  EGRVlv_rSens : Inport  Tag=%  Port=2
  EGRVlv_rOfsLrnFrst_MR : Inport  Tag=%  Port=3
  EGRVlv_rOfsLrnLst_MR : Inport  Tag=%  Port=4
  DSM_bEGRVlvReplVal : Inport  Tag=%  Port=5
  EGRVlv_rActUnCor : Inport  Tag=%  Port=6
  Add : Sum  SaturateOnIntegerOverflow=on
  Add1 : Sum  SaturateOnIntegerOverflow=on
  Add3 : Sum  SaturateOnIntegerOverflow=on
  Constant2 : Constant  Value=EGRVlv_rCmpNewCtlUn_C  SampleTime=-1
  Constant3 : Constant  Value=EGRVlv_swtActOfs_C  SampleTime=-1
  Constant4 : Constant  Value=EGRVlv_rActOfs_C  SampleTime=-1
  Logical Operator1 : Logic  Operator=OR  AllPortsSameDT=off  OutDataTypeStr=boolean
  Relational Operator1 : RelationalOperator  Operator===  OutDataTypeStr=boolean  RndMeth=Simplest
  Switch : Switch  Criteria=u2 ~= 0
  Switch1 : Switch  Criteria=u2 ~= 0
  EGRVlv_rLinOfs_mp : Outport
  EGRVlv_rActNoErrHdl : Outport  Port=2
  wires:
  EGRVlv_rSens/1 -> Add3/2
  EGRVlv_rTmpOfs/1 -> Add/2
  Switch/1 -> EGRVlv_rLinOfs_mp/1  "EGRVlv_rLinOfs_mp"
  Add3/1 -> EGRVlv_rActNoErrHdl/1
  DSM_bEGRVlvReplVal/1 -> Switch/2
  Constant2/1 -> Relational Operator1/2
  EGRVlv_rOfsLrnFrst_MR/1 -> Relational Operator1/1
  Relational Operator1/1 -> Logical Operator1/1
  Constant3/1 -> Logical Operator1/2
  Logical Operator1/1 -> Switch1/2
  EGRVlv_rOfsLrnLst_MR/1 -> Switch1/3
  Constant4/1 -> Switch1/1
  Add1/1 -> Add/1, Add3/1  "EGRVlv_rOfs_mp"
  Add/1 -> Switch/1
  Switch1/1 -> Add1/1
  EGRVlv_rActUnCor/1 -> Add1/2, Switch/3

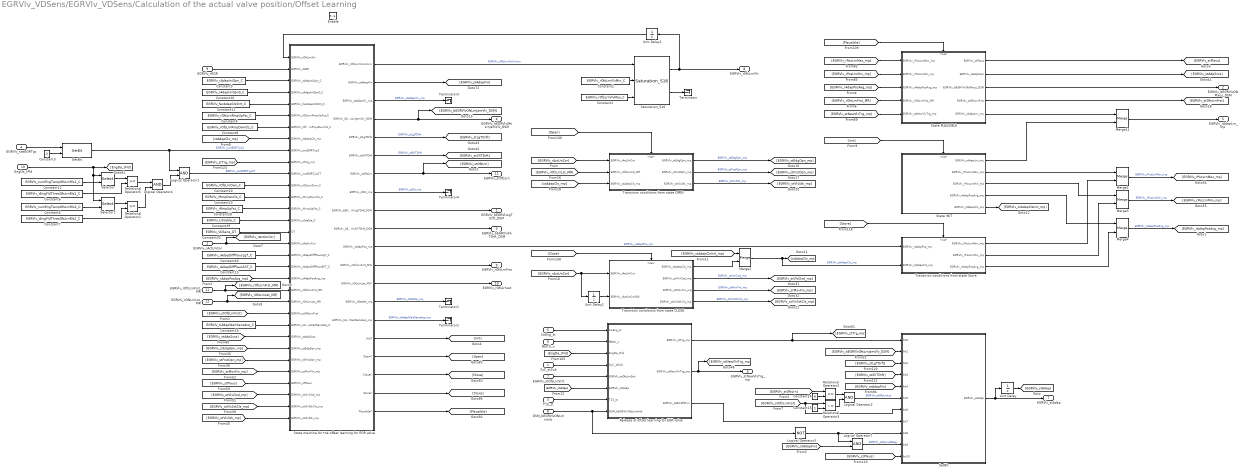
== system EGRVlv_VDSens/EGRVlv_VDSens/Calculation of the actual valve position/Offset Learning ==
  SyC_stSub : Inport  Tag=%
  EGRVlv_rActUnCor : Inport  Tag=%  Port=2
  T15_st : Inport  Tag=%  Port=3
  EGRVlv_swtEGRTyp : Inport  Tag=%  Port=4
  CoEng_st : Inport  Port=5
  BattU_u : Inport  Tag=%  Port=6
  EGRVlv_stOfsLrnStrt : Inport  Tag=%  Port=7
  DSM_bEGRVlvOfsLrnInhib : Inport  Port=8
  EGRVlv_rEGR : Inport  Tag=%  Port=9
  EngDa_tFld : Inport  Tag=%  Port=10
  EGRVlv_rOfsLrnFrst_MR : Inport  Tag=%  Port=11
  EGRVlv_rOfsLrnLst_MR : Inport  Tag=%  Port=12
  Enable : EnablePort
  Constant1 : Constant  Value=EGRVlv_rOfsLrnVlvMax_C
  Constant10 : Constant  Value=EGRVlv_rAdapIniOpn0_C
  Constant11 : Constant  Value=EGRVlv_facAdapClsStrt_C
  Constant12 : Constant  Value=EGRVlv_numEngTempOfsLrnRls1_C
  Constant13 : Constant  Value=EGRVlv_rAdapDiffPlausShT_C  SampleTime=-1
  Constant14 : Constant  Value=6  OutDataTypeStr=State_uint8
  Constant15 : Constant  OutDataTypeStr=State_uint8
  Constant16 : Constant  Value=EGRVlv_tiAdapWaitSensAcq_C  SampleTime=-1
  Constant2 : Constant  Value=EGRVlv_rOfsLrnVlvMin_C
  Constant20 : Constant  Value=EGRVlv_rOfsLrnDwn_C
  Constant23 : Constant  Value=EGRVlv_rRmpDwnCls_C
  Constant28 : Constant  Value=EGRVlv_rRmpUpFst_C
  Constant29 : Constant  Value=EGRVlv_tiStable_C
  Constant3 : Constant  Value=2  OutDataTypeStr=uint8
  Constant30 : Constant  Value=EGRVlv_VDSens_DT
  Constant4 : Constant  Value=EGRVlv_rOfsLrnRmpUpFst_C
  Constant40 : Constant  Value=EGRVlv_rAdapDiffPlausLgT_C  SampleTime=-1
  Constant5 : Constant  Value=EGRVlv_numEngTempOfsLrnRls2_C
  Constant6 : Constant  Value=EGRVlv_tEngFldThresOfsLrnRls1_C
  Constant7 : Constant  Value=EGRVlv_tEngFldThresOfsLrnRls2_C
  Constant8 : Constant  Value=EGRVlv_rOfsLrnRmpDwnCls_C
  Constant9 : Constant  Value=EGRVlv_rAdapIniOpn_C
  GetBit : CXLib/GetBit  dataTypeString=uint8  dataLength=0
      settings: AttributesFormatString=Get bit from %<dataTypeString>
  Logical Operator{1..2,4,7} (4 alike) : Logic  AllPortsSameDT=off  OutDataTypeStr=boolean
  Logical Operator3 : Logic  Operator=NOT  AllPortsSameDT=off  OutDataTypeStr=boolean
  Merge{1..4,11} (5 alike) : Merge
  Relational Operator1 : RelationalOperator  OutDataTypeStr=boolean  RndMeth=Simplest
  Relational Operator2 : RelationalOperator  Operator===  OutDataTypeStr=boolean  RndMeth=Simplest
  Relational Operator3 : RelationalOperator  Operator=~=  OutDataTypeStr=boolean  RndMeth=Simplest
  Relational Operator5 : RelationalOperator  OutDataTypeStr=boolean  RndMeth=Simplest
  Release of offset learning for EGR valve : Subsystem
  Saturation_S16 : CXLib/Saturation_S16
  Selector : Selector  IndexMode=Zero-based  InputPortWidth=3  IndexOptions=Index vector (port)  Indices=[1 3]  OutputSizes=1
  Selector1 : Selector  IndexMode=Zero-based  InputPortWidth=3  IndexOptions=Index vector (port)  Indices=[1 3]  OutputSizes=1
  SetBit : Subsystem
  State INIT : Subsystem  TreatAsAtomicUnit=on
  State PLAUSIBLE : Subsystem  TreatAsAtomicUnit=on
  State machine for the offset learning for EGR valve : Stateflow chart  TreatAsAtomicUnit=on
  Terminator{,1..4} (5 alike) : Terminator
  Transition conditions from state CLOSE : Subsystem  TreatAsAtomicUnit=on
  Transition conditions from state OPEN : Subsystem  TreatAsAtomicUnit=on
  Transition conditions from state Store : Subsystem
  Unit Delay : UnitDelay  SampleTime=-1
  Unit Delay1 : UnitDelay  SampleTime=-1
  Unit Delay2 : UnitDelay  SampleTime=-1
      settings: AttributesFormatString=InitialValue=%<InitialCondition>
  EGRVlv_bEGRVlvLgTDrft_DSM : Outport
  EGRVlv_bEGRVlvOfsPlaus_DSM : Outport  Port=2
  EGRVlv_bEGRVlvShTDrft_DSM : Outport  Port=3
  EGRVlv_bEGRVlvOfsLrnJamVlv_DSM : Outport  Tag=%  Port=4
  EGRVlv_rAdapLrn_mp : Outport  Tag=%  Port=5
  EGRVlv_stNewVlvTrg_mp : Outport  Port=6
  EGRVlv_stAdap : Outport  Port=7
  EGRVlv_rOfsLrnVlv : Outport  Port=8
  EGRVlv_rOfsLrnFrst : Outport  Port=9
  EGRVlv_rOfsLrnLst : Outport  Port=10
  EGRVlv_stOfsLrn : Outport  Tag=%  Port=11
  wires:
  Release of offset learning for EGR valve/1(EGRVlv_stTrg_mp) -> [EGRVlv_stTrg_mp], SetBit/1(bit0)
  Constant2/1 -> Saturation_S16/2
  Release of offset learning for EGR valve/3(EGRVlv_stBrkAftRun) -> SetBit/8(bit7)
  Merge11/1 -> EGRVlv_rAdapLrn_mp/1
  Release of offset learning for EGR valve/2(EGRVlv_stNewVlvTrg_mp) -> EGRVlv_stNewVlvTrg_mp/1, [EGRVlv_stNewVlvTrg_mp]
  Saturation_S16/1 -> EGRVlv_rOfsLrnVlv/1, Unit Delay1/1
  Constant1/1 -> Saturation_S16/3
  Constant5/1 -> Selector1/2
  Relational Operator5/1 -> Logical Operator4/1
  Logical Operator1/1 -> State machine for the offset learning for EGR valve/11(EGRVlv_swtEGRTyp2T)  "EGRVlv_swtEGRTyp2T"
  Logical Operator4/1 -> Logical Operator1/2
  Relational Operator1/1 -> Logical Operator4/2
  EGRVlv_rActUnCor/1 -> State machine for the offset learning for EGR valve/17(EGRVlv_rActUnCor), [EGRVlv_rActUnCor]
  Constant12/1 -> Selector/2
  EngDa_tFld/1 -> [EngDa_tFld], Selector/1, Selector1/1
  GetBit/1 -> State machine for the offset learning for EGR valve/9(EGRVlv_swtEGRTyp2), Logical Operator1/1  "EGRVlv_swtEGRTyp2"
  SetBit/1(EGRVlv_stAdap) -> EGRVlv_stAdap/1, Unit Delay/1
  Constant3/1 -> GetBit/2
  Selector/1 -> Relational Operator5/1
  State PLAUSIBLE/5(EGRVlv_rAdapLrn_mp) -> Merge11/1
  Constant7/1 -> Relational Operator1/2
  Constant6/1 -> Relational Operator5/2
  State INIT/1(EGRVlv_rAdapLrn_mp) -> Merge11/2
  Selector1/1 -> Relational Operator1/1
  [EGRVlv_stTrg_mp] -> State machine for the offset learning for EGR valve/10(EGRVlv_stTrg_mp)
  State machine for the offset learning for EGR valve/1(EGRVlv_rOfsLrnVlvUnLim) -> Saturation_S16/1  "EGRVlv_rOfsLrnVlvUnLim"
  Unit Delay/1 -> [EGRVlv_stAdap]
  [EGRVlv_stVlvStk_mp] -> State machine for the offset learning for EGR valve/32(EGRVlv_stVlvStk_mp)
  EGRVlv_swtEGRTyp/1 -> GetBit/1
  [EGRVlv_bEGRVlvOfsLrnJamVlv_DSM] -> SetBit/2(bit1)
  [EGRVlv_stLgTDrft] -> SetBit/3(bit2)
  [EGRVlv_stShTDrft] -> SetBit/4(bit3)
  [EGRVlv_stAdapFin] -> SetBit/5(bit4)
  Logical Operator2/1 -> SetBit/6(bit5)  "EGRVlv_stOfsLrnLst"
  Logical Operator7/1 -> SetBit/10(bit9)  "EGRVlv_stOpnLdDiag"
  [EGRVlv_stPlaus] -> SetBit/11(bit10)
  [EGRVlv_rPosLrnMax_mp] -> State PLAUSIBLE/1(EGRVlv_rPosLrnMax_mp)
  [EGRVlv_rPosLrnMin_mp] -> State PLAUSIBLE/2(EGRVlv_rPosLrnMin_mp)
  [EGRVlv_rAdapPosAvg_mp] -> State PLAUSIBLE/3(EGRVlv_rAdapPosAvg_mp)
  [EGRVlv_rOfsLrnFrst_MR] -> State PLAUSIBLE/4(EGRVlv_rOfsLrnFrst_MR)
  [EGRVlv_stNewVlvTrg_mp] -> State PLAUSIBLE/5(EGRVlv_stNewVlvTrg_mp)
  [Plausible] -> State PLAUSIBLE/Trigger
  [EGRVlv_rActUnCor] -> Unit Delay2/1, Transition conditions from state CLOSE/1(EGRVlv_rActUnCor)
  [Close] -> Transition conditions from state CLOSE/Trigger
  [EGRVlv_rOfsLrnLst_MR] -> Transition conditions from state OPEN/2(EGRVlv_rOfsLrnLst_MR)
  [ctAdapCls_mp] -> Transition conditions from state OPEN/3(EGRVlv_ctAdapCls_mp)
  [Open] -> Transition conditions from state OPEN/Trigger
  [Store] -> Transition conditions from state Store/Trigger
  Saturation_S16/2 -> Terminator/1
  State machine for the offset learning for EGR valve/9(EGRVlv_bEGRVlvLgTDrft_DSM) -> EGRVlv_bEGRVlvLgTDrft_DSM/1
  State PLAUSIBLE/3(EGRVlv_bEGRVlvOfsPlaus_DSM) -> EGRVlv_bEGRVlvOfsPlaus_DSM/1
  State machine for the offset learning for EGR valve/10(EGRVlv_bEGRVlvShTDrft_DSM) -> EGRVlv_bEGRVlvShTDrft_DSM/1
  State machine for the offset learning for EGR valve/3(EGRVlv_stAdapVlv_mp) -> Terminator3/1  "EGRVlv_stAdapVlv_mp"
  State machine for the offset learning for EGR valve/14(EGRVlv_tiStable_mp) -> Terminator1/1  "EGRVlv_tiStable_mp"
  State machine for the offset learning for EGR valve/11(EGRVlv_rAdapPos_mp) -> Transition conditions from state Store/1(EGRVlv_rAdapPos_mp)  "EGRVlv_rAdapPos_mp"
  State PLAUSIBLE/4(EGRVlv_stOfsLrnFrst) -> [EGRVlv_stOfsLrnFrst]
  Constant11/1 -> State machine for the offset learning for EGR valve/5(EGRVlv_facAdapClsStrt_C)
  Constant10/1 -> State machine for the offset learning for EGR valve/4(EGRVlv_rAdapIniOpn0_C)
  Constant9/1 -> State machine for the offset learning for EGR valve/3(EGRVlv_rAdapIniOpn_C)
  EGRVlv_rEGR/1 -> State machine for the offset learning for EGR valve/2(EGRVlv_rEGR)
  [EGRVlv_stVlvClsd_mp] -> State machine for the offset learning for EGR valve/30(EGRVlv_stVlvClsd_mp)
  [EGRVlv_stVlvStkCls_mp] -> State machine for the offset learning for EGR valve/31(EGRVlv_stVlvStkCls_mp)
  Constant8/1 -> State machine for the offset learning for EGR valve/7(EGRVlv_rOfsLrnRmpDwnCls_C)
  [EGRVlv_stMovFin_mp] -> State machine for the offset learning for EGR valve/28(EGRVlv_stMovFin_mp)
  Constant4/1 -> State machine for the offset learning for EGR valve/6(EGRVlv_rOfsLrnRmpUpFst_C)
  [EGRVlv_stFrstOpn_mp] -> State machine for the offset learning for EGR valve/27(EGRVlv_stFrstOpn_mp)
  [EGRVlv_stAdpSccs] -> State machine for the offset learning for EGR valve/25(EGRVlv_stAdpSccs)
  [EGRVlv_stEdgOpn_mp] -> State machine for the offset learning for EGR valve/26(EGRVlv_stEdgOpn_mp)
  [EGRVlv_stPlaus] -> State machine for the offset learning for EGR valve/29(EGRVlv_stPlaus)
  Constant20/1 -> State machine for the offset learning for EGR valve/12(EGRVlv_rOfsLrnDwn_C)
  Constant23/1 -> State machine for the offset learning for EGR valve/13(EGRVlv_rRmpDwnCls_C)
  Constant28/1 -> State machine for the offset learning for EGR valve/14(EGRVlv_rRmpUpFst_C)
  Constant29/1 -> State machine for the offset learning for EGR valve/15(EGRVlv_tiStable_C)
  Constant30/1 -> State machine for the offset learning for EGR valve/16(DT)
  [EGRVlv_stOfsLrnFrst] -> State machine for the offset learning for EGR valve/23(EGRVlv_stOfsLrnFrst)
  State machine for the offset learning for EGR valve/4(EGRVlv_bEGRVlvOfsLrnJamVlv_DSM) -> [EGRVlv_bEGRVlvOfsLrnJamVlv_DSM], EGRVlv_bEGRVlvOfsLrnJamVlv_DSM/1
  State machine for the offset learning for EGR valve/5(EGRVlv_stLgTDrft) -> [EGRVlv_stLgTDrft]  "EGRVlv_stLgTDrft"
  State machine for the offset learning for EGR valve/6(EGRVlv_stShTDrft) -> [EGRVlv_stShTDrft]  "EGRVlv_stShTDrft"
  State machine for the offset learning for EGR valve/7(EGRVlv_stOfsLrn) -> [EGRVlv_stOfsLrn], EGRVlv_stOfsLrn/1
  State machine for the offset learning for EGR valve/8(EGRVlv_stStr_mp) -> Terminator4/1  "EGRVlv_stStr_mp"
  State machine for the offset learning for EGR valve/2(EGRVlv_stAdapFin) -> [EGRVlv_stAdapFin]
  [EGRVlv_rActUnCor] -> Transition conditions from state OPEN/1(EGRVlv_rActUnCor)
  EGRVlv_rOfsLrnLst_MR/1 -> State machine for the offset learning for EGR valve/22(EGRVlv_rOfsLrnLst_MR), [EGRVlv_rOfsLrnLst_MR]
  EGRVlv_rOfsLrnFrst_MR/1 -> State machine for the offset learning for EGR valve/21(EGRVlv_rOfsLrnFrst_MR), [EGRVlv_rOfsLrnFrst_MR]
  [EGRVlv_rAdapPosAvg_mp] -> State machine for the offset learning for EGR valve/20(EGRVlv_rAdapPosAvg_mp)
  Constant13/1 -> State machine for the offset learning for EGR valve/19(EGRVlv_rAdapDiffPlausShT_C)
  Constant40/1 -> State machine for the offset learning for EGR valve/18(EGRVlv_rAdapDiffPlausLgT_C)
  State machine for the offset learning for EGR valve/13(EGRVlv_rOfsLrnLst_MW) -> EGRVlv_rOfsLrnLst/1
  State machine for the offset learning for EGR valve/15(EGRVlv_tiAdapWaitSensAcq_mp) -> Terminator2/1  "EGRVlv_tiAdapWaitSensAcq_mp"
  [EGRVlv_stAdapFin] -> Logical Operator7/2
  [EGRVlv_stOfsLrn] -> Relational Operator2/1
  Constant14/1 -> Relational Operator2/2
  [EGRVlv_stOfsLrnFrst] -> SetBit/7(bit6), Relational Operator3/1
  Constant15/1 -> Relational Operator3/2
  Relational Operator2/1 -> Logical Operator2/1
  Relational Operator3/1 -> Logical Operator2/2
  Constant16/1 -> State machine for the offset learning for EGR valve/24(EGRVlv_tiAdapWaitSensAcq_C)
  Logical Operator3/1 -> Logical Operator7/1, SetBit/9(bit8)
  Unit Delay1/1 -> State machine for the offset learning for EGR valve/1(EGRVlv_rOfsLrnVlv)
  [ctAdapCls_mp] -> State machine for the offset learning for EGR valve/8(EGRVlv_ctAdapCls_mp)
  Merge2/1 -> [EGRVlv_rPosLrnMax_mp]  "EGRVlv_rPosLrnMax_mp"
  Merge3/1 -> [EGRVlv_rPosLrnMin_mp]  "EGRVlv_rPosLrnMin_mp"
  Merge4/1 -> [EGRVlv_rAdapPosAvg_mp]  "EGRVlv_rAdapPosAvg_mp"
  State machine for the offset learning for EGR valve/17(Open()) -> [Open]
  State machine for the offset learning for EGR valve/18(Close()) -> [Close]
  State machine for the offset learning for EGR valve/19(Store()) -> [Store]
  State machine for the offset learning for EGR valve/20(Plausible()) -> [Plausible]
  Transition conditions from state OPEN/2(EGRVlv_stFrstOpn_mp) -> [EGRVlv_stFrstOpn_mp]  "EGRVlv_stFrstOpn_mp"
  Transition conditions from state OPEN/1(EGRVlv_stEdgOpn_mp) -> [EGRVlv_stEdgOpn_mp]  "EGRVlv_stEdgOpn_mp"
  Transition conditions from state OPEN/3(EGRVlv_stVlvStk_mp) -> [EGRVlv_stVlvStk_mp]  "EGRVlv_stVlvStk_mp"
  Transition conditions from state CLOSE/2(EGRVlv_stVlvClsd_mp) -> [EGRVlv_stVlvClsd_mp]  "EGRVlv_stVlvClsd_mp"
  Transition conditions from state CLOSE/3(EGRVlv_stMovFin_mp) -> [EGRVlv_stMovFin_mp]  "EGRVlv_stMovFin_mp"
  Transition conditions from state CLOSE/4(EGRVlv_stVlvStkCls_mp) -> [EGRVlv_stVlvStkCls_mp]  "EGRVlv_stVlvStkCls_mp"
  State PLAUSIBLE/2(EGRVlv_stAdpSccs) -> [EGRVlv_stAdpSccs]
  State machine for the offset learning for EGR valve/16(Init()) -> [Init]
  [Init] -> State INIT/Trigger
  Merge1/1 -> Transition conditions from state Store/2(EGRVlv_ctAdapCls_mp), [ctAdapCls_mp]  "EGRVlv_ctAdapCls_mp"
  Transition conditions from state CLOSE/1(EGRVlv_ctAdapCls_mp) -> Merge1/2
  State INIT/2(EGRVlv_rPosLrnMax_mp) -> Merge2/1
  State INIT/3(EGRVlv_rPosLrnMin_mp) -> Merge3/1
  State INIT/4(EGRVlv_rAdapPosAvg_mp) -> Merge4/1
  State INIT/5(EGRVlv_ctAdapCls_mp) -> [EGRVlv_ctAdapClsInit_mp]
  [EGRVlv_ctAdapClsInit_mp] -> Merge1/1
  Transition conditions from state Store/1(EGRVlv_rPosLrnMax_mp) -> Merge2/2
  Transition conditions from state Store/2(EGRVlv_rPosLrnMin_mp) -> Merge3/2
  Transition conditions from state Store/3(EGRVlv_rAdapPosAvg_mp) -> Merge4/2
  Unit Delay2/1 -> Transition conditions from state CLOSE/2(EGRVlv_rActUnCorOld)
  State PLAUSIBLE/1(EGRVlv_stPlaus) -> [EGRVlv_stPlaus]
  DSM_bEGRVlvOfsLrnInhib/1 -> Logical Operator3/1, Release of offset learning for EGR valve/8(DSM_bEGRVlvOfsLrnInhib)
  CoEng_st/1 -> Release of offset learning for EGR valve/1(CoEng_st)
  BattU_u/1 -> Release of offset learning for EGR valve/2(BattU_u)
  [EngDa_tFld] -> Release of offset learning for EGR valve/3(EngDa_tFld)
  SyC_stSub/1 -> Release of offset learning for EGR valve/4(SyC_stSub)
  EGRVlv_stOfsLrnStrt/1 -> Release of offset learning for EGR valve/5(EGRVlv_stOfsLrnStrt)
  [EGRVlv_stAdap] -> Release of offset learning for EGR valve/6(EGRVlv_stAdap)
  T15_st/1 -> Release of offset learning for EGR valve/7(T15_st)
  State machine for the offset learning for EGR valve/12(EGRVlv_rOfsLrnFrst_MW) -> EGRVlv_rOfsLrnFrst/1

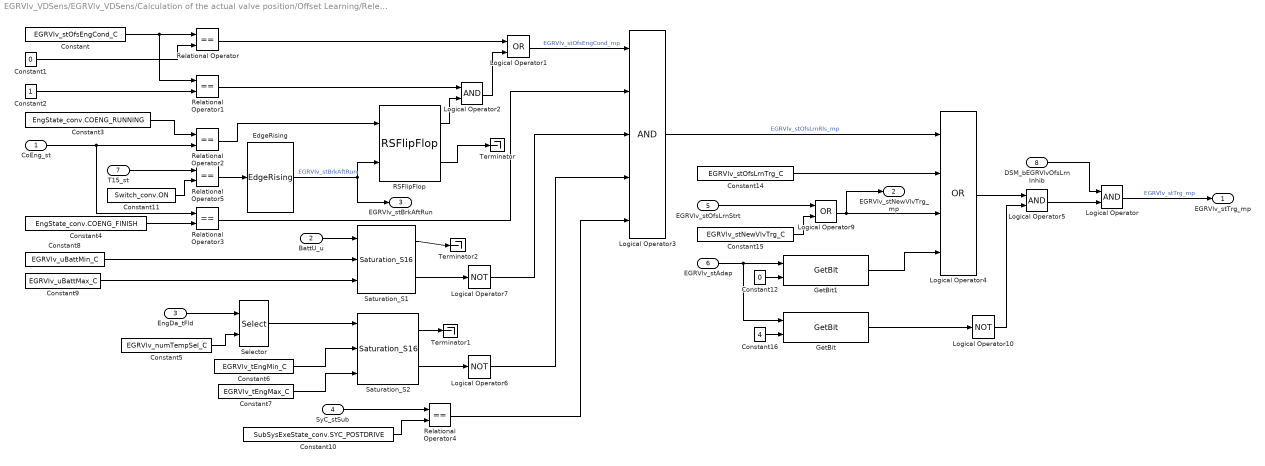
== system EGRVlv_VDSens/EGRVlv_VDSens/Calculation of the actual valve position/Offset Learning/Release of offset learning for EGR valve ==
  CoEng_st : Inport
  BattU_u : Inport  Tag=%  Port=2
  EngDa_tFld : Inport  Tag=%  Port=3
  SyC_stSub : Inport  Tag=%  Port=4
  EGRVlv_stOfsLrnStrt : Inport  Tag=%  Port=5
  EGRVlv_stAdap : Inport  Tag=%  Port=6
  T15_st : Inport  Tag=%  Port=7
  DSM_bEGRVlvOfsLrnInhib : Inport  Port=8
  Constant : Constant  Value=EGRVlv_stOfsEngCond_C
  Constant1 : Constant  Value=0  OutDataTypeStr=boolean
  Constant10 : Constant  Value=SubSysExeState_conv.SYC_POSTDRIVE  OutDataTypeStr=Enum:SubSysExeState_conv
  Constant11 : Constant  Value=Switch_conv.ON
  Constant12 : Constant  Value=0  OutDataTypeStr=uint8
  Constant14 : Constant  Value=EGRVlv_stOfsLrnTrg_C  SampleTime=-1
  Constant15 : Constant  Value=EGRVlv_stNewVlvTrg_C  SampleTime=-1
  Constant16 : Constant  Value=4  OutDataTypeStr=uint8
  Constant2 : Constant  OutDataTypeStr=boolean
  Constant3 : Constant  Value=EngState_conv.COENG_RUNNING
  Constant4 : Constant  Value=EngState_conv.COENG_FINISH
  Constant5 : Constant  Value=EGRVlv_numTempSel_C  SampleTime=-1
  Constant6 : Constant  Value=EGRVlv_tEngMin_C  SampleTime=-1
  Constant7 : Constant  Value=EGRVlv_tEngMax_C  SampleTime=-1
  Constant8 : Constant  Value=EGRVlv_uBattMin_C  SampleTime=-1
  Constant9 : Constant  Value=EGRVlv_uBattMax_C  SampleTime=-1
  EdgeRising : CXLib/EdgeRising
  GetBit : CXLib/GetBit  dataTypeString=uint16  dataLength=0
      settings: AttributesFormatString=Get bit from %<dataTypeString>
  GetBit1 : CXLib/GetBit  dataTypeString=uint16  dataLength=0
      settings: AttributesFormatString=Get bit from %<dataTypeString>
  Logical Operator : Logic  AllPortsSameDT=off  OutDataTypeStr=boolean
  Logical Operator1 : Logic  Operator=OR  AllPortsSameDT=off  OutDataTypeStr=boolean
  Logical Operator10 : Logic  Operator=NOT  AllPortsSameDT=off  OutDataTypeStr=boolean
  Logical Operator2 : Logic  AllPortsSameDT=off  OutDataTypeStr=boolean
  Logical Operator3 : Logic  Inputs=5  AllPortsSameDT=off  OutDataTypeStr=boolean
  Logical Operator4 : Logic  Operator=OR  Inputs=4  AllPortsSameDT=off  OutDataTypeStr=boolean
  Logical Operator5 : Logic  AllPortsSameDT=off  OutDataTypeStr=boolean
  Logical Operator6 : Logic  Operator=NOT  AllPortsSameDT=off  OutDataTypeStr=boolean
  Logical Operator7 : Logic  Operator=NOT  AllPortsSameDT=off  OutDataTypeStr=boolean
  Logical Operator9 : Logic  Operator=OR  AllPortsSameDT=off  OutDataTypeStr=boolean
  RSFlipFlop : CXLib/RSFlipFlop
  Relational Operator{,1..5} (6 alike) : RelationalOperator  Operator===  OutDataTypeStr=boolean  RndMeth=Simplest
  Saturation_S1 : CXLib/Saturation_S16
  Saturation_S2 : CXLib/Saturation_S16
  Selector : Selector  IndexMode=Zero-based  InputPortWidth=3  IndexOptions=Index vector (port)  Indices=[1 3]  OutputSizes=1
  Terminator : Terminator
  Terminator1 : Terminator
  Terminator2 : Terminator
  EGRVlv_stTrg_mp : Outport
  EGRVlv_stNewVlvTrg_mp : Outport  Port=2
  EGRVlv_stBrkAftRun : Outport  Port=3
  wires:
  Logical Operator/1 -> EGRVlv_stTrg_mp/1  "EGRVlv_stTrg_mp"
  DSM_bEGRVlvOfsLrnInhib/1 -> Logical Operator/1
  Constant/1 -> Relational Operator/1, Relational Operator1/1
  Constant1/1 -> Relational Operator/2
  Relational Operator/1 -> Logical Operator1/1
  Constant2/1 -> Relational Operator1/2
  Relational Operator1/1 -> Logical Operator2/1
  Logical Operator2/1 -> Logical Operator1/2
  Constant3/1 -> Relational Operator2/1
  Relational Operator2/1 -> RSFlipFlop/1
  RSFlipFlop/1 -> Logical Operator2/2
  CoEng_st/1 -> Relational Operator3/1, Relational Operator2/2
  Constant4/1 -> Relational Operator3/2
  Logical Operator1/1 -> Logical Operator3/1  "EGRVlv_stOfsEngCond_mp"
  Relational Operator3/1 -> Logical Operator3/2
  Logical Operator3/1 -> Logical Operator4/1  "EGRVlv_stOfsLrnRls_mp"
  Logical Operator4/1 -> Logical Operator5/1
  Logical Operator5/1 -> Logical Operator/2
  Saturation_S2/2 -> Logical Operator6/1
  Logical Operator6/1 -> Logical Operator3/4
  Constant5/1 -> Selector/2
  EngDa_tFld/1 -> Selector/1
  Selector/1 -> Saturation_S2/1
  Constant6/1 -> Saturation_S2/2
  Constant7/1 -> Saturation_S2/3
  Saturation_S1/2 -> Logical Operator7/1
  Constant8/1 -> Saturation_S1/2
  Constant9/1 -> Saturation_S1/3
  Logical Operator7/1 -> Logical Operator3/3
  Constant10/1 -> Relational Operator4/2
  SyC_stSub/1 -> Relational Operator4/1
  Relational Operator4/1 -> Logical Operator3/5
  Constant15/1 -> Logical Operator9/2
  EGRVlv_stOfsLrnStrt/1 -> Logical Operator9/1
  Constant14/1 -> Logical Operator4/2
  Logical Operator9/1 -> Logical Operator4/3, EGRVlv_stNewVlvTrg_mp/1
  Constant16/1 -> GetBit/2
  GetBit/1 -> Logical Operator10/1
  Logical Operator10/1 -> Logical Operator5/2
  EdgeRising/1 -> RSFlipFlop/2, EGRVlv_stBrkAftRun/1  "EGRVlv_stBrkAftRun"
  T15_st/1 -> Relational Operator5/1
  Relational Operator5/1 -> EdgeRising/1
  Constant11/1 -> Relational Operator5/2
  BattU_u/1 -> Saturation_S1/1
  RSFlipFlop/2 -> Terminator/1
  Saturation_S1/1 -> Terminator2/1
  Saturation_S2/1 -> Terminator1/1
  Constant12/1 -> GetBit1/2
  EGRVlv_stAdap/1 -> GetBit1/1, GetBit/1
  GetBit1/1 -> Logical Operator4/4
